simulink model "Nonlinear_model"  (R2022b)
settings: Solver=ode45  StartTime=0.0  StopTime=10  RelTol=1e-3
undefined symbols (not defined in the file or in its folder): u1
settings Model: Creator=henrr  LastModifiedBy=henrr
settings DataIOCC: SaveOutput=off  SaveTime=off  ReturnWorkspaceOutputs=off

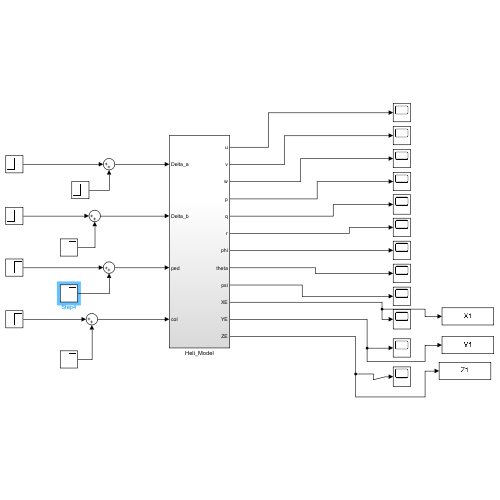
[thumbnail: Simulink's stored preview of the top-level diagram]
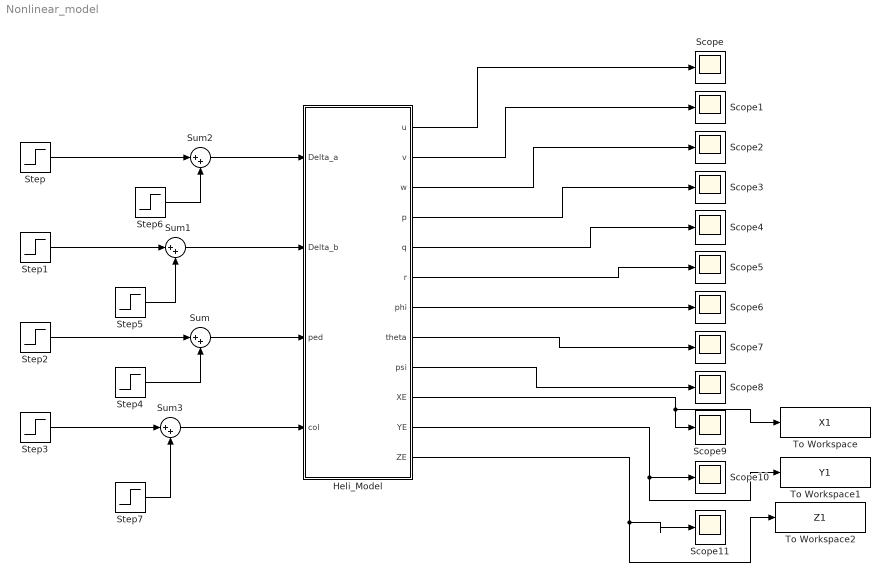
== system Nonlinear_model ==
  Heli_Model : Subsystem
  Scope{,1..11} (12 alike) : Scope
  Step : Step  Time=0  Before=u1(1)  After=u1(1)  SampleTime=0
  Step1 : Step  Time=0  Before=u1(2)  After=u1(2)  SampleTime=0
  Step2 : Step  Time=0  Before=u1(3)  After=u1(3)  SampleTime=0
  Step3 : Step  Time=0  Before=u1(4)  After=u1(4)  SampleTime=0
  Step4 : Step  Time=0  SampleTime=0
  Step5 : Step  Time=0  After=0  SampleTime=0
  Step6 : Step  Time=0  After=0  SampleTime=0
  Step7 : Step  Time=0  After=0  SampleTime=0
  Sum{,1..3} (4 alike) : Sum  Inputs=|++
  To Workspace : ToWorkspace  VariableName=X1  SaveFormat=Timeseries  SampleTime=-1
  To Workspace1 : ToWorkspace  VariableName=Y1  SaveFormat=Timeseries  SampleTime=-1
  To Workspace2 : ToWorkspace  VariableName=Z1  SaveFormat=Timeseries  SampleTime=-1
  wires:
  Heli_Model/1(u) -> Scope/1
  Heli_Model/2(v) -> Scope1/1
  Heli_Model/3(w) -> Scope2/1
  Heli_Model/4(p) -> Scope3/1
  Heli_Model/5(q) -> Scope4/1
  Heli_Model/6(r) -> Scope5/1
  Heli_Model/7(phi) -> Scope6/1
  Heli_Model/8(theta) -> Scope7/1
  Heli_Model/9(psi) -> Scope8/1
  Heli_Model/10(XE) -> Scope9/1, To Workspace/1
  Heli_Model/11(YE) -> To Workspace1/1, Scope10/1
  Heli_Model/12(ZE) -> To Workspace2/1, Scope11/1
  Step2/1 -> Sum/1
  Step4/1 -> Sum/2
  Sum/1 -> Heli_Model/3(ped)
  Sum1/1 -> Heli_Model/2(Delta_b)
  Step1/1 -> Sum1/1
  Step5/1 -> Sum1/2
  Sum2/1 -> Heli_Model/1(Delta_a)
  Step/1 -> Sum2/1
  Step6/1 -> Sum2/2
  Sum3/1 -> Heli_Model/4(col)
  Step3/1 -> Sum3/1
  Step7/1 -> Sum3/2

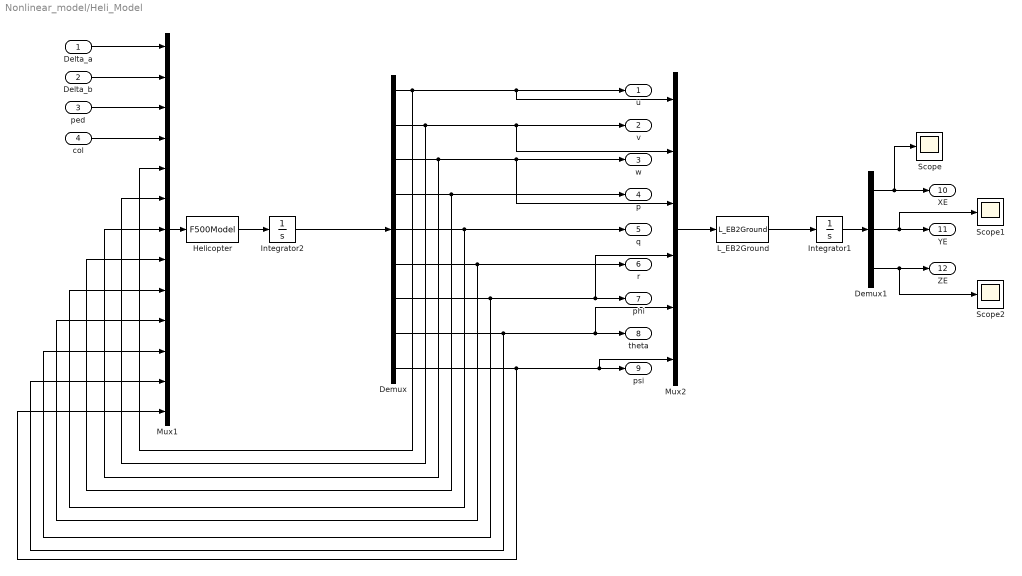
== system Nonlinear_model/Heli_Model ==
  Delta_a : Inport
  Delta_b : Inport  Port=2
  ped : Inport  Port=3
  col : Inport  Port=4
  Demux : Demux  Outputs=9
  Demux1 : Demux  Outputs=3
  Helicopter : MATLABFcn  MATLABFcn=F500Model
  Integrator1 : Integrator  InitialCondition=[20 10 20]
  Integrator2 : Integrator  InitialCondition=[0 0 0 0 0 0 0 0 0]
  L_EB2Ground : MATLABFcn  MATLABFcn=L_EB2Ground
  Mux1 : Mux  Inputs=13
  Mux2 : Mux  Inputs=6
  Scope : Scope
  Scope1 : Scope
  Scope2 : Scope
  u : Outport
  v : Outport  Port=2
  w : Outport  Port=3
  p : Outport  Port=4
  q : Outport  Port=5
  r : Outport  Port=6
  phi : Outport  Port=7
  theta : Outport  Port=8
  psi : Outport  Port=9
  XE : Outport  Port=10
  YE : Outport  Port=11
  ZE : Outport  Port=12
  wires:
  Demux/1 -> Mux1/5, u/1, Mux2/1
  Demux/2 -> Mux1/6, v/1, Mux2/2
  Demux/3 -> Mux1/7, w/1, Mux2/3
  Demux/4 -> Mux1/8, p/1
  Demux/5 -> Mux1/9, q/1
  Demux/6 -> Mux1/10, r/1
  Demux/7 -> Mux1/11, phi/1, Mux2/4
  Demux/8 -> Mux1/12, theta/1, Mux2/5
  Demux/9 -> Mux1/13, psi/1, Mux2/6
  Demux1/1 -> XE/1, Scope/1
  Demux1/2 -> YE/1, Scope1/1
  Demux1/3 -> ZE/1, Scope2/1
  Mux2/1 -> L_EB2Ground/1
  L_EB2Ground/1 -> Integrator1/1
  Integrator1/1 -> Demux1/1
  Mux1/1 -> Helicopter/1
  col/1 -> Mux1/4
  Integrator2/1 -> Demux/1
  ped/1 -> Mux1/3
  Delta_a/1 -> Mux1/1
  Delta_b/1 -> Mux1/2
  Helicopter/1 -> Integrator2/1
